simulink model "model"  (R2023b)
settings: Solver=VariableStepAuto  StartTime=0.0  StopTime=30  FixedStep=0.0001  RelTol=1e-6  AbsTol=1e-6  EnableMultiTasking=on
undefined symbols (not defined in the file or in its folder): init
settings Model: Creator=pmorin  LastModifiedBy=haoyuan
settings SolverCC: AutoScaleAbsTol=off  AlgebraicLoopSolver=TrustRegion
settings DataIOCC: LimitDataPoints=on  SaveFormat=Array  SignalLoggingSaveFormat=ModelDataLogs  ReturnWorkspaceOutputs=off
settings OptimizationCC: BooleanDataType=off  ExpressionDepthLimit=2147483647  LifeSpan=inf
settings DebuggingCC: SaveWithParameterizedLinksMsg=none  UnderspecifiedInitializationDetection=Classic  MergeDetectMultiDrivingBlocksExec=none  SignalResolutionControl=TryResolveAllWithWarning  MultiTaskDSMMsg=warning  MultiTaskCondExecSysMsg=none  FcnCallInpInsideContextMsg=warning  UnconnectedInputMsg=warning  UnconnectedOutputMsg=warning  UnconnectedLineMsg=warning  StateNameClashWarn=warning  SFUnexpectedBacktrackingDiag=warning  SFNoUnconditionalDefaultTransitionDiag=warning  SFExecutionAtInitializationDiag=none  ArithmeticOperatorsInVariantConditions=warning
settings HardwareCC: ProdBitPerPointer=32  ProdBitPerSizeT=32  ProdBitPerPtrDiffT=32  ProdLargestAtomicFloat=None  ProdIntDivRoundTo=Undefined  ProdEndianess=Unspecified  ProdWordSize=32  ProdHWDeviceType=32-bit Generic  TargetUnknown=on
settings ModelReferenceCC: EnableRefExpFcnMdlSchedulingChecks=on  PropagateSignalLabelsOutOfModel=off
settings SFSimCC: SimUseLocalCustomCode=off  CustomCodeUndefinedFunction=UseInterfaceOnly
settings RTWCC: RTWUseLocalCustomCode=off
settings CodeAppCC: StateflowObjectComments=on
settings GRTTargetCC: TargetLangStandard=C89/C90 (ANSI)  CombineOutputUpdateFcns=off  GRTInterface=on
settings ConfigComp: CovMetricSettings=dw  CovSaveCumulativeToWorkspaceVar=on  CovSaveSingleToWorkspaceVar=on  CovExternalEMLEnable=off

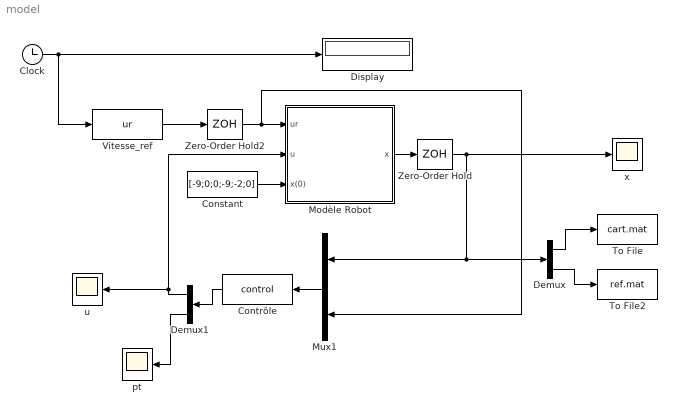
== system model ==
  Clock : Clock
  Constant : Constant  Value=[-9;0;0;-9;-2;0]
  Contrôle : MATLABFcn  MATLABFcn=control  OutputDimensions=4
  Demux : Demux  Outputs=[3;3]
  Demux1 : Demux  Outputs=[2;2]
  Display : Display
  Modèle Robot : Subsystem
  Mux1 : Mux  Inputs=2
  To File : ToFile  Filename=cart.mat
  To File2 : ToFile  Filename=ref.mat
  "Vitesse_ref " : MATLABFcn  MATLABFcn=ur  OutputDimensions=2
  Zero-Order Hold : ZeroOrderHold  SampleTime=0.01
  Zero-Order Hold2 : ZeroOrderHold  SampleTime=0.01
  pt : Scope
  u : Scope
  x : Scope
  wires:
  Mux1/1 -> Contrôle/1
  Constant/1 -> Modèle Robot/3(x(0))
  Modèle Robot/1(x) -> Zero-Order Hold/1
  Zero-Order Hold/1 -> x/1, Demux/1, Mux1/1
  Clock/1 -> "Vitesse_ref "/1, Display/1
  Zero-Order Hold2/1 -> Mux1/2, Modèle Robot/1(ur)
  "Vitesse_ref "/1 -> Zero-Order Hold2/1
  Demux/1 -> To File/1
  Demux/2 -> To File2/1
  Contrôle/1 -> Demux1/1
  Demux1/1 -> u/1, Modèle Robot/2(u)
  Demux1/2 -> pt/1

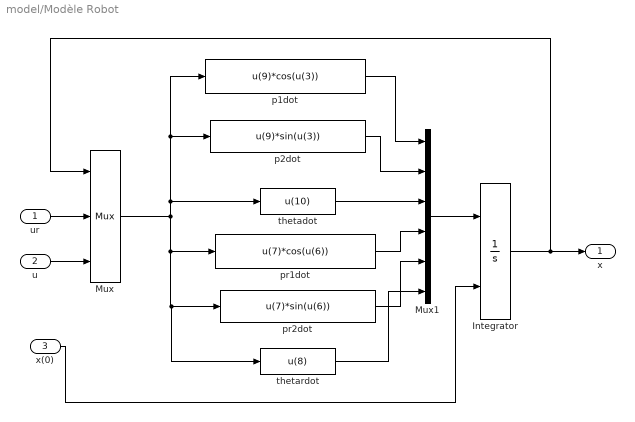
== system model/Modèle Robot ==
  ur : Inport
  u : Inport  Port=2
  x(0) : Inport  Port=3
  Integrator : Integrator  InitialConditionSource=external  InitialCondition=init
  Mux : Mux  Inputs=[6 2 2]
  Mux1 : Mux  Inputs=6
  p1dot : Fcn  Expr=u(9)*cos(u(3))
  p2dot : Fcn  Expr=u(9)*sin(u(3))
  pr1dot : Fcn  Expr=u(7)*cos(u(6))
  pr2dot : Fcn  Expr=u(7)*sin(u(6))
  thetadot : Fcn  Expr=u(10)
  thetardot : Fcn  Expr=u(8)
  x : Outport
  wires:
  Integrator/1 -> x/1, Mux/1
  Mux1/1 -> Integrator/1
  p1dot/1 -> Mux1/1
  thetadot/1 -> Mux1/3
  Mux/1 -> thetardot/1, pr2dot/1, pr1dot/1, p1dot/1, p2dot/1, thetadot/1
  p2dot/1 -> Mux1/2
  x(0)/1 -> Integrator/2
  u/1 -> Mux/3
  ur/1 -> Mux/2
  pr1dot/1 -> Mux1/4
  pr2dot/1 -> Mux1/5
  thetardot/1 -> Mux1/6
